simulink library "metux_library"  (R2025b)
settings: Solver=VariableStepAuto  StartTime=0.0  StopTime=10.0  RelTol=1e-3
values from neighbouring files (symbols this model uses):
  controllerGains = Simulink.Parameter(controllerGains)    [currentControllerInit.m]
  R = 287    [fluid_contants.m]
undefined symbols (not defined in the file or in its folder): b, bp, bv, DiscIntNeverNeededParam, fluid, Fs_max, J, Km, kp, L, omega_bandwidth, T_brk, T_c, valveAngle, valveFit
libraries: simulink x5, slpidlib x1, eeGeneralControl x1
settings Model: Creator=karadeli  LastModifiedBy=karadeli

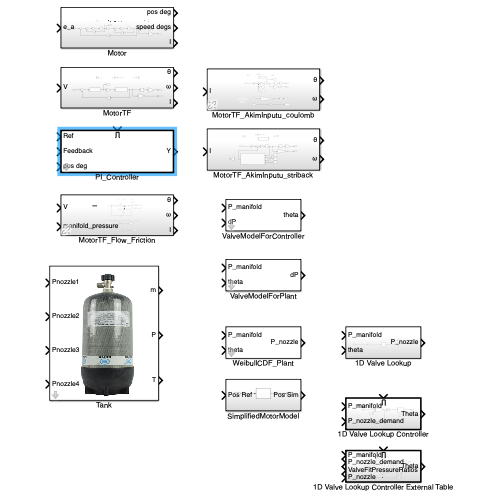
[thumbnail: Simulink's stored preview of the top-level diagram]
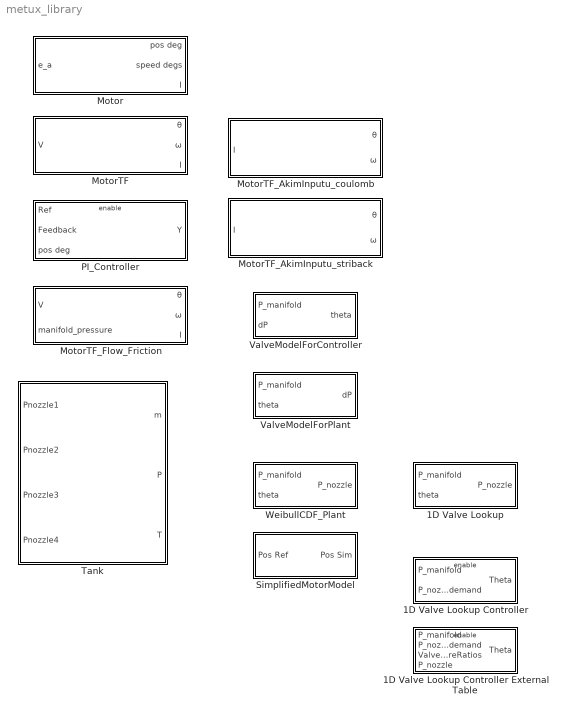
== system metux_library ==
  1D Valve Lookup : Subsystem
  1D Valve Lookup Controller : Subsystem
  1D Valve Lookup Controller External Table : Subsystem
  Motor : Subsystem
  MotorTF : Subsystem
  MotorTF_AkimInputu_coulomb : Subsystem  AncestorBlock=metux_library/MotorTF
  MotorTF_AkimInputu_striback : Subsystem
  MotorTF_Flow_Friction : Subsystem  AncestorBlock=metux_library/MotorTF
  PI_Controller : Subsystem  mask{Kp=1, Ki=1, SatMax=0, SatMin=0, Ts=1e-3, RateLimiterMax=0, RateLimiterMin=0}
  SimplifiedMotorModel : Subsystem
  Tank : Subsystem  mask{P0=300, T0=25, mdotGain=fluid.mdotGain, V=fluid.V, R=fluid.R, Cv=fluid.Cv, Patm=fluid.Patm}
      mask Display: image('Tank.png');
  ValveModelForController : Subsystem  mask{alpha=51.8534, C_max=0.9197}
  ValveModelForPlant : Subsystem  mask{C_max=0.9197, alpha=51.8534}
  WeibullCDF_Plant : Subsystem  mask{L=0.7772, tau=519.6652, n=1.5198}

== system metux_library/1D Valve Lookup ==
  P_manifold : Inport  Unit=psi
  theta : Inport  Port=2  Unit=deg
  1-D Lookup Table : Lookup_n-D  NumberOfTableDimensions=1  BreakpointsForDimension1=valveFit.angles  Table=valveFit.pressureRatios  InterpMethod=Linear Lagrange  ExtrapMethod=Clip  InternalRulePriority=Speed  RndMeth=Simplest
  Product1 : Product
  Saturation : Saturate  UpperLimit=5*360  LowerLimit=0
  P_nozzle : Outport  Unit=psi
  wires:
  1-D Lookup Table/1 -> Product1/2
  P_manifold/1 -> Product1/1
  Product1/1 -> P_nozzle/1
  theta/1 -> Saturation/1
  Saturation/1 -> 1-D Lookup Table/1

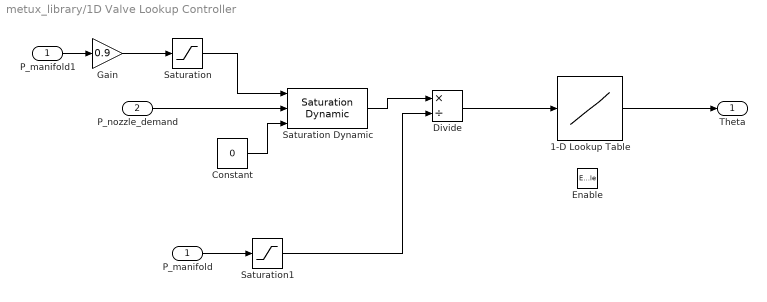
== system metux_library/1D Valve Lookup Controller ==
  P_manifold : Inport  Unit=psi
  P_nozzle_demand : Inport  Port=2  Unit=psi
  Enable : EnablePort
  1-D Lookup Table : Lookup_n-D  NumberOfTableDimensions=1  BreakpointsForDimension1=valveFit.pressureRatios  Table=valveFit.angles  InterpMethod=Linear Lagrange  ExtrapMethod=Clip  InternalRulePriority=Speed  RndMeth=Simplest
  Constant : Constant  Value=0
  Divide : Product  Inputs=*/
  Gain : Gain  Gain=0.9
  P_manifold1 : InportShadow  Unit=psi
  Saturation : Saturate  UpperLimit=5000  LowerLimit=15
  Saturation Dynamic : simulink/Discontinuities/Saturation Dynamic  OutMin=[]  OutMax=[]  OutDataTypeStr=Inherit: Same as second input  OutDataType=fixdt(1, 16)  OutScaling=2^-10  DoSatur=off
  Saturation1 : Saturate  UpperLimit=5000  LowerLimit=15
  Theta : Outport  Unit=deg
  wires:
  P_nozzle_demand/1 -> Saturation Dynamic/2
  1-D Lookup Table/1 -> Theta/1
  Saturation Dynamic/1 -> Divide/1
  Constant/1 -> Saturation Dynamic/3
  P_manifold1/1 -> Gain/1
  Gain/1 -> Saturation/1
  Saturation/1 -> Saturation Dynamic/1
  P_manifold/1 -> Saturation1/1
  Saturation1/1 -> Divide/2
  Divide/1 -> 1-D Lookup Table/1

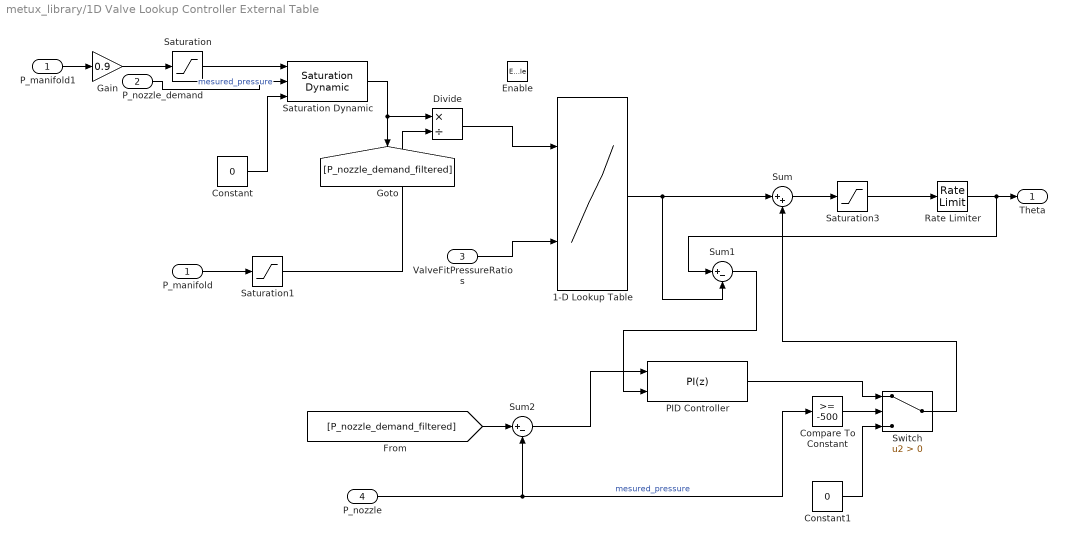
== system metux_library/1D Valve Lookup Controller External Table ==
  P_manifold : Inport  Unit=psi
  P_nozzle_demand : Inport  Port=2  Unit=psi
  ValveFitPressureRatios : Inport  Port=3  Unit=psi  PortDimensions=11
  P_nozzle : Inport  Port=4
  Enable : EnablePort
  1-D Lookup Table : Lookup_n-D  NumberOfTableDimensions=1  BreakpointsForDimension1Source=Input port  BreakpointsForDimension1=valveFit.pressureRatios  Table=[0 100 200 300 400 500 600 800 900 1100 1200 ]  InterpMethod=Linear Lagrange  ExtrapMethod=Clip  InternalRulePriority=Speed  RndMeth=Simplest
      settings: InputPortMap=u0,p5
  Compare To Constant : simulink/Logic and Bit Operations/Compare To Constant  relop=>=  const=-500  OutDataTypeStr=boolean
  Constant : Constant  Value=0
  Constant1 : Constant  Value=0
  Divide : Product  Inputs=*/
  Gain : Gain  Gain=0.9
  PID Controller : slpidlib/PID Controller  Controller=PI  Form=Parallel  TimeDomain=Discrete-time  UseExternalTs=off  SampleTime=-1  IntegratorMethod=Forward Euler  FilterMethod=Forward Euler  ControllerParametersSource=internal  P=controllerGains.pressure.Kp  I=controllerGains.pressure.Ki  UseKiTs=off  D=0  UseExternalDerivativeSource=off  N=100  UseFilter=on  TunerSelectOption=Transfer Function Based (PID Tuner App)  InitialConditionSource=internal  InitialConditionForIntegrator=0  InitialConditionForFilter=0  DifferentiatorICPrevScaledInput=0  ExternalReset=none  TrackingMode=on  Kt=100  LimitOutput=off  SatLimitsSource=internal  UpperSaturationLimit=200  LowerSaturationLimit=-200  LinearizeAsGain=on  AntiWindupMode=none  Kb=1  LimitIntegrator=off  UpperIntegratorSaturationLimit=200  LowerIntegratorSaturationLimit=-200  POutMin=[]  POutMax=[]  IOutMin=[]  IOutMax=[]  DOutMin=[]  DOutMax=[]  NOutMin=[]  NOutMax=[]  SumOutMin=[]  SumOutMax=[]  SaturationOutMin=[]  SaturationOutMax=[]  PParamMin=[]  PParamMax=[]  IParamMin=[]  IParamMax=[]  DParamMin=[]  DParamMax=[]  NParamMin=[]  NParamMax=[]  KbParamMin=[]  KbParamMax=[]  KtParamMin=[]  KtParamMax=[]  KbOutMin=[]  KbOutMax=[]  KtOutMin=[]  KtOutMax=[]  IntegratorOutMin=[]  IntegratorOutMax=[]  FilterOutMin=[]  FilterOutMax=[]  SumI1OutMin=[]  SumI1OutMax=[]  SumI2OutMin=[]  SumI2OutMax=[]  SumI3OutMin=[]  SumI3OutMax=[]  SumI4OutMin=[]  SumI4OutMax=[]  SumDOutMin=[]  SumDOutMax=[]  DifferentiatorOutMin=[]  DifferentiatorOutMax=[]  FilterDiffOutCoefMin=[]  FilterDiffOutCoefMax=[]  ReciprocalOutMin=[]  ReciprocalOutMax=[]  SumDenOutMin=[]  SumDenOutMax=[]  SumNumOutMin=[]  SumNumOutMax=[]  DivideOutMin=[]  DivideOutMax=[]  UdiffTsProdOutMin=[]  UdiffTsProdOutMax=[]  NTsProdOutMin=[]  NTsProdOutMax=[]  UintegralTsProdOutMin=[]  UintegralTsProdOutMax=[]  UngainTsProdOutMin=[]  UngainTsProdOutMax=[]  ClampingZeroOutDataTypeStr=Inherit: Inherit via back propagation  ClampingZeroOutMin=[]  ClampingZeroOutMax=[]  FilterDenConstantOutDataTypeStr=Inherit: Inherit via back propagation  FilterDenConstantOutMin=[]  FilterDenConstantOutMax=[]  PCopyOutDataTypeStr=Inherit: Inherit via back propagation  PCopyOutMin=[]  PCopyOutMax=[]  NCopyOutDataTypeStr=Inherit: Inherit via back propagation  NCopyOutMin=[]  NCopyOutMax=[]  IntegratorContinuousStateAttributes=''  IntegratorStateMustResolveToSignalObject=off  IntegratorRTWStateStorageClass=Auto  FilterContinuousStateAttributes=''  FilterStateMustResolveToSignalObject=off  FilterRTWStateStorageClass=Auto  ParallelPVariant=InternalParameters  IdealPVariant=Disabled  IVariant=InternalParameters  DVariant=Disabled  IntegratorVariant=Discrete  SatVariant=Disabled  AWVariant=Passthrough  PCopyVariant=Disabled  TRVariant=Enabled  FdbkBlocksVariant=Forward  IdealPFdbkVariant=Disabled  SatFdbkVariant=Disabled  DerivativeFilterVariant=Disabled  NVariant=Disabled  NCopyVariant=Disabled_SignalSpec  FilterICVariant=Disabled  IntegratorICVariant=InternalICs  ExternalResetVariant=Disabled  TRSumVariant=TrackingMode  SumFdbkVariant=Disabled  SumVariant=Sum_PI  TsampFilterVariant=InternalTs  TsampNgainVariant=Passthrough  TsampIntegralVariant=Disabled_SignalSpec  ExternalSaturationOutDataTypeStr=Inherit: Same as second input  DerivativeSourceVariant=Disabled  PreIntVariant=InternalPreInt
  P_manifold1 : InportShadow  Unit=psi
  Rate Limiter : RateLimiter  RisingSlewLimit=2000  FallingSlewLimit=-2000  SampleTimeMode=inherited
  Saturation : Saturate  UpperLimit=5000  LowerLimit=15
  Saturation Dynamic : simulink/Discontinuities/Saturation Dynamic  OutMin=[]  OutMax=[]  OutDataTypeStr=Inherit: Same as second input  OutDataType=fixdt(1, 16)  OutScaling=2^-10  DoSatur=off
  Saturation1 : Saturate  UpperLimit=5000  LowerLimit=15
  Saturation3 : Saturate  UpperLimit=1200  LowerLimit=0
  Sum : Sum  Inputs=|++
  Sum1 : Sum  Inputs=|+-
  Sum2 : Sum  Inputs=|+-
  Switch : Switch  Criteria=u2 > Threshold  SaturateOnIntegerOverflow=off  InputSameDT=off
  Theta : Outport  Unit=deg
  wires:
  Divide/1 -> 1-D Lookup Table/1
  Saturation1/1 -> Divide/2
  P_manifold/1 -> Saturation1/1
  Saturation/1 -> Saturation Dynamic/1
  Gain/1 -> Saturation/1
  P_manifold1/1 -> Gain/1
  Constant/1 -> Saturation Dynamic/3
  1-D Lookup Table/1 -> Sum1/2, Sum/1
  P_nozzle_demand/1 -> Saturation Dynamic/2  "mesured_pressure"
  ValveFitPressureRatios/1 -> 1-D Lookup Table/2
  P_nozzle/1 -> Compare To Constant/1, Sum2/2  "mesured_pressure"
  Saturation Dynamic/1 -> [P_nozzle_demand_filtered], Divide/1
  Sum2/1 -> PID Controller/1
  Saturation3/1 -> Rate Limiter/1
  Sum/1 -> Saturation3/1
  Switch/1 -> Sum/2
  Compare To Constant/1 -> Switch/2
  PID Controller/1 -> Switch/1
  Constant1/1 -> Switch/3
  [P_nozzle_demand_filtered] -> Sum2/1
  Rate Limiter/1 -> Sum1/1, Theta/1
  Sum1/1 -> PID Controller/2

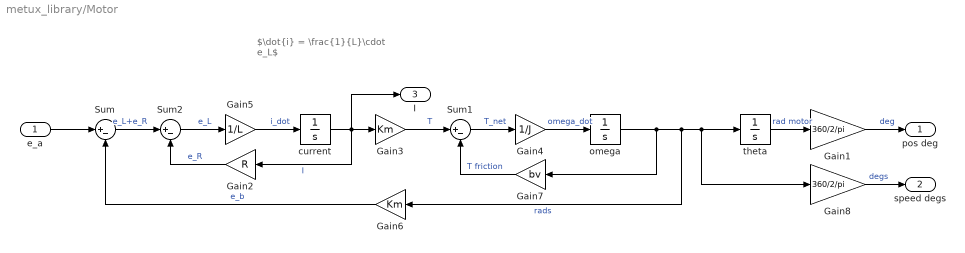
== system metux_library/Motor ==
  note: $\dot{i} = \frac{1}{L}\cdot e_L$
  e_a : Inport
  Gain1 : Gain  Gain=360/2/pi
  Gain2 : Gain  Gain=R
  Gain3 : Gain  Gain=Km
  Gain4 : Gain  Gain=1/J
  Gain5 : Gain  Gain=1/L
  Gain6 : Gain  Gain=Km
  Gain7 : Gain  Gain=bv
  Gain8 : Gain  Gain=360/2/pi
  Sum : Sum  Inputs=|+-
  Sum1 : Sum  Inputs=|+-
  Sum2 : Sum  Inputs=|+-
  current : Integrator
  omega : Integrator
  theta : Integrator  InitialCondition=valveAngle.Data(1)*13.7/180*pi  ZeroCross=off
  pos deg : Outport
  speed degs : Outport  Port=2
  I : Outport  Port=3
  wires:
  Sum1/1 -> Gain4/1  "T_net"
  theta/1 -> Gain1/1  "rad motor"
  current/1 -> Gain3/1, Gain2/1, I/1  "I"
  Sum/1 -> Sum2/1  "e_L+e_R"
  Gain5/1 -> current/1  "i_dot"
  Gain4/1 -> omega/1  "omega_dot"
  Gain2/1 -> Sum2/2  "e_R"
  Gain3/1 -> Sum1/1  "T"
  Gain6/1 -> Sum/2  "e_b"
  Gain7/1 -> Sum1/2  "T friction"
  Sum2/1 -> Gain5/1  "e_L"
  omega/1 -> theta/1, Gain8/1, Gain6/1, Gain7/1  "rads"
  e_a/1 -> Sum/1
  Gain1/1 -> pos deg/1  "deg"
  Gain8/1 -> speed degs/1  "degs"

== system metux_library/MotorTF ==
  note: $e_b = K_b\cdot\frac{d\theta}{dt}$
  note: $L_a\cdot\frac{di_a}{dt}+R_ai_a+e_b=e_a$
  note: $\frac{di}{dt} = \frac{1}{L}\cdot e_L$
  V : Inport  Unit=V
  Gain1 : Gain  Gain=360/2/pi
  Gain3 : Gain  Gain=Km
  Gain6 : Gain  Gain=Km
  Gain8 : Gain  Gain=360/2/pi
  Sum : Sum  Inputs=|+-
  current : TransferFcn  Denominator=[L R]  ContinuousStateAttributes='current'
  speed : TransferFcn  Denominator=[J bv]  ContinuousStateAttributes='speed'
  theta : Integrator  ZeroCross=off
  θ : Outport  Unit=deg
  ω : Outport  Port=2  Unit=deg/s
  I : Outport  Port=3  Unit=A
  wires:
  Gain1/1 -> θ/1  "deg"
  theta/1 -> Gain1/1  "rad motor"
  Gain8/1 -> ω/1  "degs"
  speed/1 -> theta/1, Gain8/1, Gain6/1  "rads"
  Gain3/1 -> speed/1  "T"
  current/1 -> Gain3/1, I/1  "I"
  Gain6/1 -> Sum/2  "e_b"
  Sum/1 -> current/1  "e_L+e_R"
  V/1 -> Sum/1

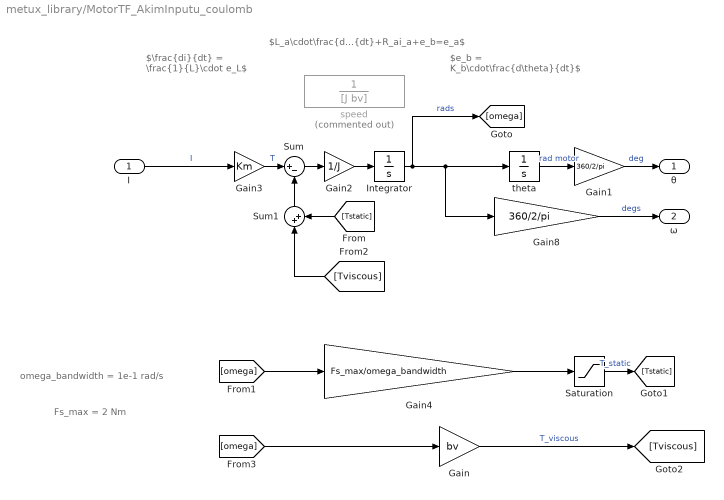
== system metux_library/MotorTF_AkimInputu_coulomb ==
  note: Fs_max = 2 Nm
  note: omega_bandwidth = 1e-1 rad/s
  note: $\frac{di}{dt} = \frac{1}{L}\cdot e_L$
  note: $L_a\cdot\frac{di_a}{dt}+R_ai_a+e_b=e_a$
  note: $e_b = K_b\cdot\frac{d\theta}{dt}$
  I : Inport  Unit=A
  Gain : Gain  Gain=bv
  Gain1 : Gain  Gain=360/2/pi
  Gain2 : Gain  Gain=1/J
  Gain3 : Gain  Gain=Km
  Gain4 : Gain  Gain=Fs_max/omega_bandwidth
  Gain8 : Gain  Gain=360/2/pi
  Integrator : Integrator
  Saturation : Saturate  UpperLimit=Fs_max  LowerLimit=-Fs_max  ZeroCross=off
  Sum : Sum  Inputs=|+-
  Sum1 : Sum  Inputs=|++
  speed : TransferFcn  Commented=on  Denominator=[J bv]  ContinuousStateAttributes='speed'
  theta : Integrator  ZeroCross=off
  θ : Outport  Unit=deg
  ω : Outport  Port=2  Unit=deg/s
  wires:
  I/1 -> Gain3/1  "I"
  Gain3/1 -> Sum/1  "T"
  Integrator/1 -> [omega], Gain8/1, theta/1  "rads"
  Gain8/1 -> ω/1  "degs"
  theta/1 -> Gain1/1  "rad motor"
  Gain1/1 -> θ/1  "deg"
  Sum/1 -> Gain2/1
  Gain2/1 -> Integrator/1
  [omega] -> Gain4/1
  Gain4/1 -> Saturation/1
  Sum1/1 -> Sum/2
  Saturation/1 -> [Tstatic]  "T_static"
  [Tstatic] -> Sum1/2
  Gain/1 -> [Tviscous]  "T_viscous"
  [Tviscous] -> Sum1/1
  [omega] -> Gain/1

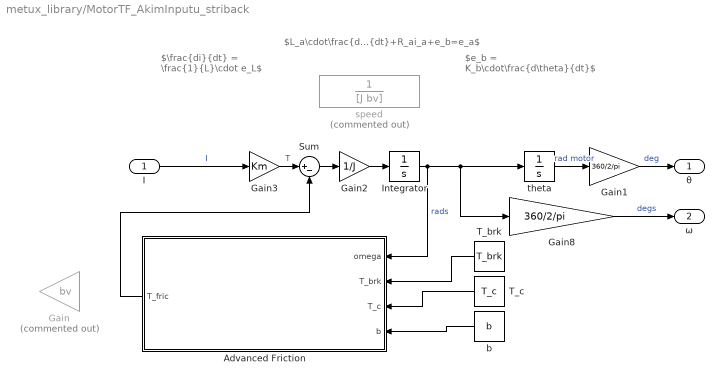
== system metux_library/MotorTF_AkimInputu_striback ==
  note: $e_b = K_b\cdot\frac{d\theta}{dt}$
  note: $L_a\cdot\frac{di_a}{dt}+R_ai_a+e_b=e_a$
  note: $\frac{di}{dt} = \frac{1}{L}\cdot e_L$
  I : Inport  Unit=A
  Advanced Friction : MATLAB Function  TreatAsAtomicUnit=on
  Gain : Gain  Commented=on  Gain=bv
  Gain1 : Gain  Gain=360/2/pi
  Gain2 : Gain  Gain=1/J
  Gain3 : Gain  Gain=Km
  Gain8 : Gain  Gain=360/2/pi
  Integrator : Integrator
  Sum : Sum  Inputs=|+-
  T_brk : Constant  Value=T_brk
  T_c : Constant  Value=T_c
  b : Constant  Value=b
  speed : TransferFcn  Commented=on  Denominator=[J bv]  ContinuousStateAttributes='speed'
  theta : Integrator  ZeroCross=off
  θ : Outport  Unit=deg
  ω : Outport  Port=2  Unit=deg/s
  wires:
  T_brk/1 -> Advanced Friction/2(T_brk)
  b/1 -> Advanced Friction/4(b)
  T_c/1 -> Advanced Friction/3(T_c)
  Gain2/1 -> Integrator/1
  Advanced Friction/1(T_fric) -> Sum/2
  Sum/1 -> Gain2/1
  Gain1/1 -> θ/1  "deg"
  theta/1 -> Gain1/1  "rad motor"
  Gain8/1 -> ω/1  "degs"
  Integrator/1 -> Advanced Friction/1(omega), theta/1, Gain8/1  "rads"
  Gain3/1 -> Sum/1  "T"
  I/1 -> Gain3/1  "I"

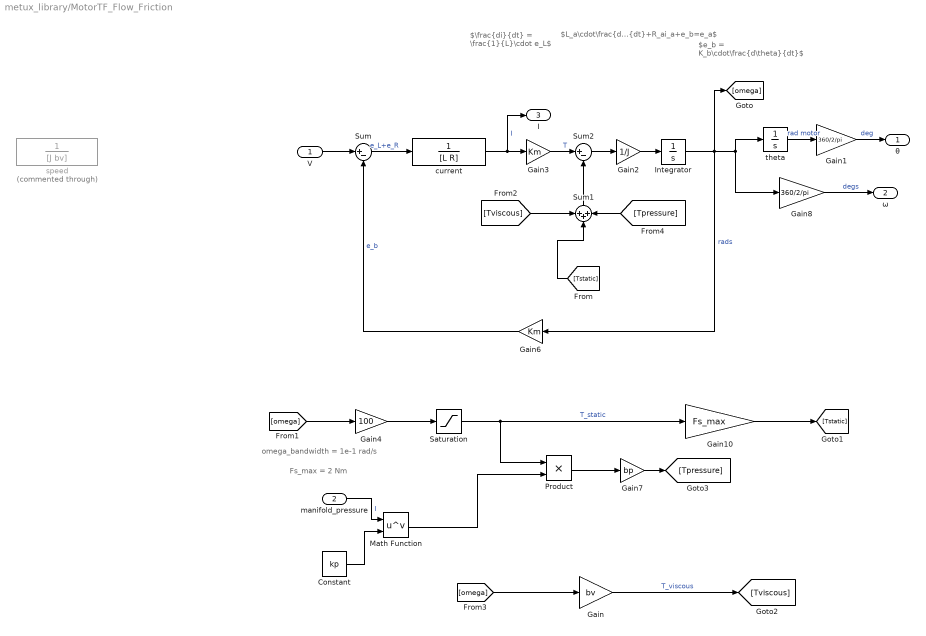
== system metux_library/MotorTF_Flow_Friction ==
  note: $\frac{di}{dt} = \frac{1}{L}\cdot e_L$
  note: $L_a\cdot\frac{di_a}{dt}+R_ai_a+e_b=e_a$
  note: $e_b = K_b\cdot\frac{d\theta}{dt}$
  note: Fs_max = 2 Nm
  note: omega_bandwidth = 1e-1 rad/s
  V : Inport  Unit=V
  manifold_pressure : Inport  Port=2
  Constant : Constant  Value=kp
  Gain : Gain  Gain=bv
  Gain1 : Gain  Gain=360/2/pi
  Gain10 : Gain  Gain=Fs_max
  Gain2 : Gain  Gain=1/J
  Gain3 : Gain  Gain=Km
  Gain4 : Gain  Gain=100
  Gain6 : Gain  Gain=Km
  Gain7 : Gain  Gain=bp
  Gain8 : Gain  Gain=360/2/pi
  Integrator : Integrator
  Math Function : Math  Operator=pow
  Product : Product
  Saturation : Saturate  UpperLimit=1  LowerLimit=-1
  Sum : Sum  Inputs=|+-
  Sum1 : Sum  Inputs=+++
  Sum2 : Sum  Inputs=|+-
  current : TransferFcn  Denominator=[L R]  ContinuousStateAttributes='current'
  speed : TransferFcn  Commented=through  Denominator=[J bv]  ContinuousStateAttributes='speed'
  theta : Integrator  ZeroCross=off
  θ : Outport  Unit=deg
  ω : Outport  Port=2  Unit=deg/s
  I : Outport  Port=3  Unit=A
  wires:
  V/1 -> Sum/1
  Sum/1 -> current/1  "e_L+e_R"
  Gain6/1 -> Sum/2  "e_b"
  current/1 -> I/1, Gain3/1  "I"
  Gain3/1 -> Sum2/1  "T"
  Integrator/1 -> Gain6/1, Gain8/1, theta/1, [omega]  "rads"
  Gain8/1 -> ω/1  "degs"
  theta/1 -> Gain1/1  "rad motor"
  Gain1/1 -> θ/1  "deg"
  [omega] -> Gain4/1
  Constant/1 -> Math Function/2
  Product/1 -> Gain7/1
  [omega] -> Gain/1
  Gain/1 -> [Tviscous]  "T_viscous"
  Saturation/1 -> Gain10/1, Product/1  "T_static"
  manifold_pressure/1 -> Math Function/1  "I"
  Gain10/1 -> [Tstatic]
  Gain7/1 -> [Tpressure]
  Math Function/1 -> Product/2
  Gain4/1 -> Saturation/1
  [Tstatic] -> Sum1/2
  [Tpressure] -> Sum1/3
  Sum1/1 -> Sum2/2
  [Tviscous] -> Sum1/1
  Sum2/1 -> Gain2/1
  Gain2/1 -> Integrator/1

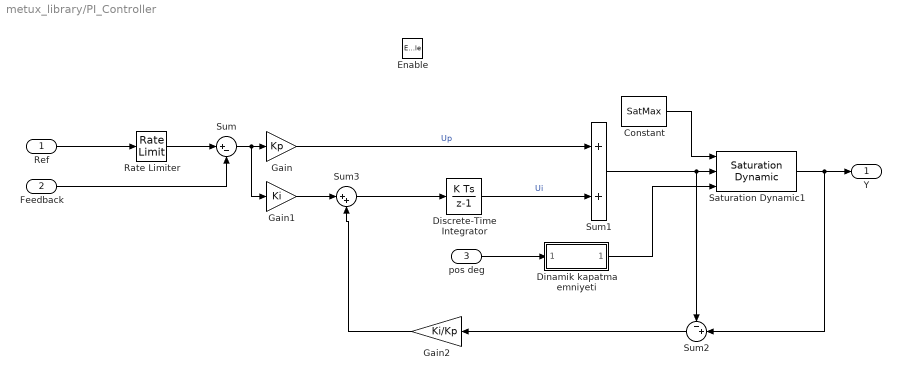
== system metux_library/PI_Controller ==
  Ref : Inport  SampleTime=Ts
  Feedback : Inport  Port=2  SampleTime=Ts
  pos deg : Inport  Port=3
  Enable : EnablePort  StatesWhenEnabling=reset
  Constant : Constant  Value=SatMax
  Dinamik kapatma emniyeti : Subsystem
  Discrete-Time Integrator : DiscreteIntegrator  SampleTime=Ts  LimitOutput=on  UpperSaturationLimit=SatMax  LowerSaturationLimit=SatMin  ICPrevOutput=DiscIntNeverNeededParam  ICPrevScaledInput=DiscIntNeverNeededParam
  Gain : Gain  Gain=Kp
  Gain1 : Gain  Gain=Ki
  Gain2 : Gain  Gain=Ki/Kp
  Rate Limiter : RateLimiter  RisingSlewLimit=RateLimiterMax  FallingSlewLimit=RateLimiterMin  SampleTimeMode=inherited
  Saturation Dynamic1 : simulink/Discontinuities/Saturation Dynamic  OutMin=[]  OutMax=[]  OutDataTypeStr=Inherit: Same as second input  OutDataType=fixdt(1, 16)  OutScaling=2^-10  DoSatur=off
  Sum : Sum  Inputs=|+-
  Sum1 : Sum
  Sum2 : Sum  Inputs=-+|
  Sum3 : Sum  Inputs=|++
  Y : Outport  SampleTime=Ts  OutputWhenDisabled=reset  InitialOutput=[0.0]
  wires:
  Saturation Dynamic1/1 -> Y/1, Sum2/2
  Discrete-Time Integrator/1 -> Sum1/2  "Ui"
  Gain1/1 -> Sum3/1
  Sum/1 -> Gain1/1, Gain/1
  Gain/1 -> Sum1/1  "Up"
  Feedback/1 -> Sum/2
  Sum1/1 -> Saturation Dynamic1/2, Sum2/1
  Ref/1 -> Rate Limiter/1
  Sum2/1 -> Gain2/1
  Gain2/1 -> Sum3/2
  Rate Limiter/1 -> Sum/1
  Constant/1 -> Saturation Dynamic1/1
  Sum3/1 -> Discrete-Time Integrator/1
  pos deg/1 -> Dinamik kapatma emniyeti/1(pos deg)
  Dinamik kapatma emniyeti/1(Lower Sat Limit) -> Saturation Dynamic1/3

== system metux_library/SimplifiedMotorModel ==
  Pos Ref : Inport  Unit=deg
  Second-Order Filter : eeGeneralControl/Second-Order Filter  FilterType=Low-pass  fn=20  Zeta=0.8  Ts=0  A0=0  Ph0=0  f0=0  b0=0
  Pos Sim : Outport  Unit=deg
  wires:
  Pos Ref/1 -> Second-Order Filter/1
  Second-Order Filter/1 -> Pos Sim/1

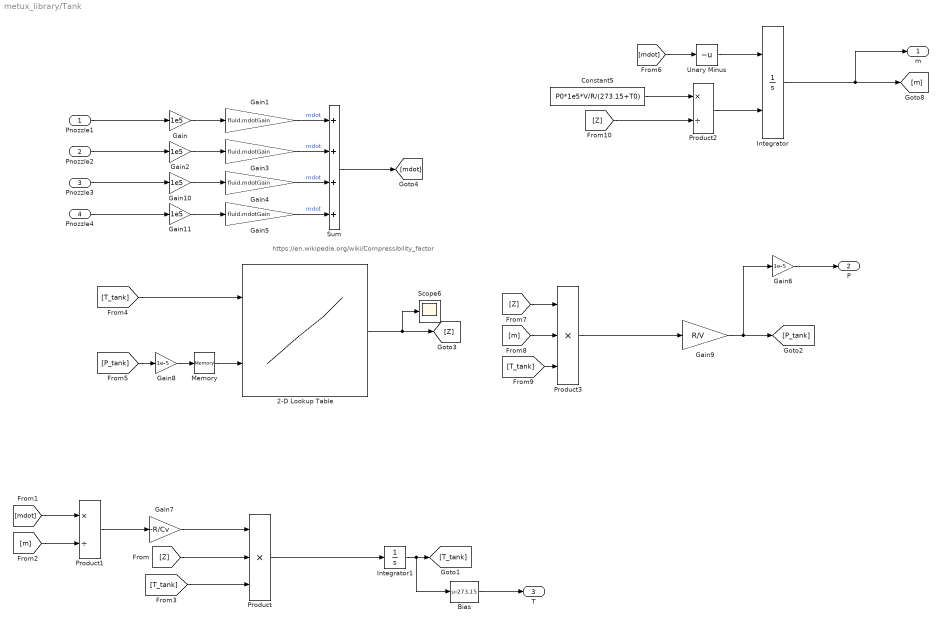
== system metux_library/Tank ==
  note: https://en.wikipedia.org/wiki/Compressibility_factor
  Pnozzle1 : Inport  Unit=bar
  Pnozzle2 : Inport  Port=2  Unit=bar
  Pnozzle3 : Inport  Port=3  Unit=bar
  Pnozzle4 : Inport  Port=4  Unit=bar
  2-D Lookup Table : Lookup_n-D  BreakpointsForDimension1=[75;80;90;100;120;140;160;180;200;250;300;350;400;450;500;600;800;1000]  BreakpointsForDimension2=[1;5;10;20;40;60;80;100;150;200;250;300;400;500]  Table=[0.0052 0.0260 0.0519 0.1036 0.2063 0.3082 0.4094 0.5099 0.7581 1.0125 0.0000 0.0000 0.0000 0.0000;0.0000 0.0250 0.0499 0.0995 0.1981 0.2958 0.3927 0.4887 0.7258 0.9588 1.1931 1.4139 0.0000 0.0000;0.9764 0.0236 0.0453 0.0940 0.1866 0.2781 0.3686 0.4681 0.6779 0.8929 1.1098 1.3110 1.7161 2.1105;0.9797 0.8872 0.0453 0.0900 0.1782 0.2635 0.3498 0.4337 0.6386 0.8377 1.0395 1.2227 1.5937 1.9536;0.9880 0.9373 0.8860 0.6730 0.1778 0.2557 0.3371 0.4132 0.5964 0.7720 0.9530 1.1076 1.5091 1.7366;0.9927 0.9614 0.9205 0.8297 0.5856 0.3313 0.3737 0.4340 0.5909 0.7699 0.9114 1.0393 1.3202 1.5903;0.9951 0.9748 0.9489 0.8954 0.7803 0.6603 0.5696 0.5489 0.6340 0.7564 0.8840 1.0105 1.2585 1.4970;0.9967 0.9832 0.9660 0.9314 0.8625 0.7977 0.7432 0.7084 0.7180 0.7986 0.9000 1.0068 1.2232 1.4361;0.9978 0.9886 0.9767 0.9539 0.9100 0.8701 0.8374 0.8142 0.8061 0.8549 0.9311 1.0185 1.2054 1.3944;0.9992 0.9957 0.9911 0.9822 0.9671 0.9549 0.9463 0.9411 0.9450 0.9713 1.0152 1.0702 1.1990 1.3392;0.9999 0.9987 0.9974 0.9950 0.9917 0.9901 0.9903 0.9930 1.0074 1.0326 1.0669 1.1089 1.2073 1.3163;1.0000 1.0002 1.0004 1.0014 1.0038 1.0075 1.0121 1.0183 1.0377 1.0635 1.0947 1.1303 1.2116 1.3015;1.0002 1.0012 1.0025 1.0046 1.0100 1.0159 1.0229 1.0312 1.0533 1.0795 1.1087 1.1411 1.2117 1.2890;1.0003 1.0016 1.0034 1.0063 1.0133 1.0210 1.0287 1.0374 1.0614 1.0913 1.1183 1.1463 1.2090 1.2778;1.0003 1.0020 1.0034 1.0074 1.0151 1.0234 1.0323 1.0410 1.0650 1.0913 1.1183 1.1463 1.2051 1.2667;1.0004 1.0022 1.0039 1.0081 1.0164 1.0253 1.0340 1.0434 1.0678 1.0920 1.1172 1.1427 1.1947 1.2475;1.0004 1.0020 1.0038 1.0077 1.0157 1.0240 1.0321 1.0408 1.0621 1.0844 1.1061 1.1283 1.1720 1.2150;1.0004 1.0018 1.0037 1.0068 1.0142 1.0215 1.0290 1.0365 1.0556 1.0744 1.0948 1.1131 1.1515 1.1889]  InternalRulePriority=Speed  RndMeth=Simplest
      settings: InputPortMap=u0,u1
  Bias : Bias  Bias=-273.15  SaturateOnIntegerOverflow=off
  Constant5 : Constant  Value=P0*1e5*V/R/(273.15+T0)
  Gain{,2,10..11} (4 alike) : Gain  Gain=1e5
  Gain{1,3..5} (4 alike) : Gain  Gain=fluid.mdotGain
  Gain6 : Gain  Gain=1e-5
  Gain7 : Gain  Gain=-R/Cv
  Gain8 : Gain  Gain=1e-5
  Gain9 : Gain  Gain=R/V
  Integrator : Integrator  InitialConditionSource=external  InitialCondition=3  LimitOutput=on  UpperSaturationLimit=5  LowerSaturationLimit=Patm*V/R/100
  Integrator1 : Integrator  InitialCondition=T0+273.15  LowerSaturationLimit=0
  Memory : Memory  InitialCondition=P0
  Product : Product  Inputs=3
  Product1 : Product  Inputs=*/
  Product2 : Product  Inputs=*/
  Product3 : Product  Inputs=3
  Scope6 : Scope
      settings: ActiveDisplayYMinimum=0.8767629134747118  ActiveDisplayYMaximum=1.1251537258363551  DataLoggingVariableName=ScopeData19
  Sum : Sum  Inputs=4
  Unary Minus : UnaryMinus
  m : Outport  Unit=kg
  P : Outport  Port=2  Unit=bar
  T : Outport  Port=3  Unit=°C
  wires:
  Gain1/1 -> Sum/1  "mdot"
  Pnozzle1/1 -> Gain/1
  Unary Minus/1 -> Integrator/1
  Integrator/1 -> m/1, [m]
  [mdot] -> Unary Minus/1
  Constant5/1 -> Product2/1
  Pnozzle2/1 -> Gain2/1
  Pnozzle3/1 -> Gain10/1
  Pnozzle4/1 -> Gain11/1
  Gain5/1 -> Sum/4  "mdot"
  Gain4/1 -> Sum/3  "mdot"
  Gain3/1 -> Sum/2  "mdot"
  Sum/1 -> [mdot]
  Bias/1 -> T/1
  Gain6/1 -> P/1
  Gain7/1 -> Product/1
  Product/1 -> Integrator1/1
  Product1/1 -> Gain7/1
  [m] -> Product1/2
  Integrator1/1 -> Bias/1, [T_tank]
  [mdot] -> Product1/1
  [Z] -> Product/2
  [T_tank] -> Product/3
  Gain8/1 -> Memory/1
  2-D Lookup Table/1 -> [Z], Scope6/1
  [T_tank] -> 2-D Lookup Table/1
  [P_tank] -> Gain8/1
  Memory/1 -> 2-D Lookup Table/2
  Product3/1 -> Gain9/1
  Gain9/1 -> Gain6/1, [P_tank]
  [Z] -> Product3/1
  [m] -> Product3/2
  [T_tank] -> Product3/3
  Product2/1 -> Integrator/2
  [Z] -> Product2/2
  Gain/1 -> Gain1/1
  Gain2/1 -> Gain3/1
  Gain10/1 -> Gain4/1
  Gain11/1 -> Gain5/1

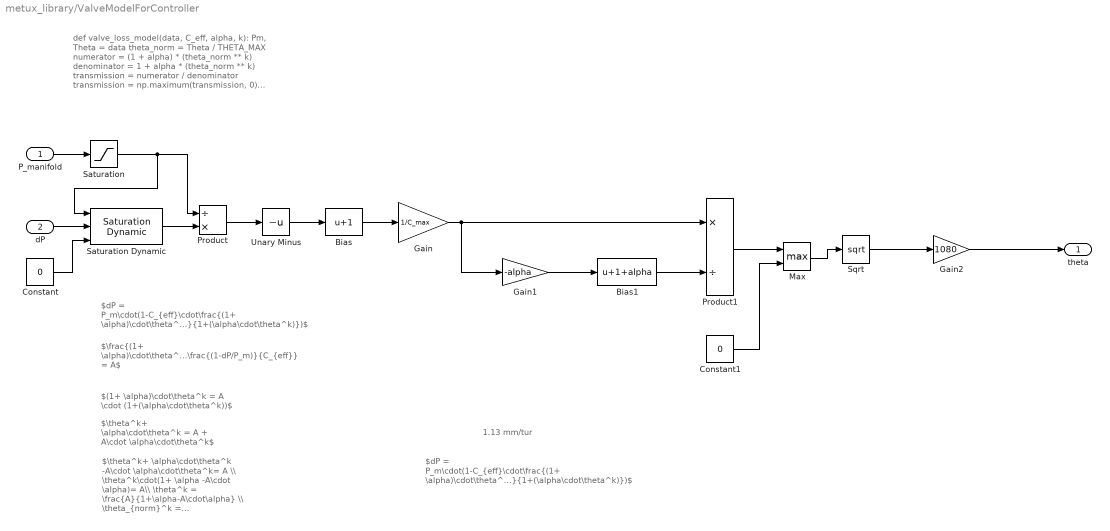
== system metux_library/ValveModelForController ==
  note: 1.13 mm/tur
  note: $dP = P_m\cdot(1-C_{eff}\cdot\frac{(1+ \alpha)\cdot\theta^k}{1+(\alpha\cdot\theta^k)})$
  note: def valve_loss_model(data, C_eff, alpha, k):
      |     Pm, Theta = data
      |     theta_norm = Theta / THETA_MAX
      |
      |     numerator = (1 + alpha) * (theta_norm ** k)
      |     denominator = 1 + alpha * (theta_norm ** k)
      |     transmission = numerator / denominator
      |     transmission = np.maximum(transmission, 0)
      |
      |     return Pm * (1 - C_eff * transmission)
  note: $\frac{(1+ \alpha)\cdot\theta^k}{1+(\alpha\cdot\theta^k)}=\frac{(1-dP/P_m)}{C_{eff}} = A$
  note: $(1+ \alpha)\cdot\theta^k = A \cdot (1+(\alpha\cdot\theta^k))$
  note: $\theta^k+ \alpha\cdot\theta^k = A + A\cdot \alpha\cdot\theta^k$
  note: $\theta^k+ \alpha\cdot\theta^k -A\cdot \alpha\cdot\theta^k= A \\ \theta^k\cdot(1+ \alpha -A\cdot \alpha)= A\\ \theta^k = \frac{A}{1+\alpha-A\cdot\alpha} \\ \theta_{norm}^k = \frac{\frac{(1-dP/P_m)}{C_{eff}}}{1+\alpha-(\frac{(1-dP/P_m)}{C_{eff}})\cdot\alpha}$
  note: $dP = P_m\cdot(1-C_{eff}\cdot\frac{(1+ \alpha)\cdot\theta^k}{1+(\alpha\cdot\theta^k)})$
  P_manifold : Inport
  dP : Inport  Port=2
  Bias : Bias  Bias=1  SaturateOnIntegerOverflow=off
  Bias1 : Bias  Bias=1+alpha  SaturateOnIntegerOverflow=off
  Constant : Constant  Value=0
  Constant1 : Constant  Value=0  OutDataTypeStr=single
  Gain : Gain  Gain=1/C_max
  Gain1 : Gain  Gain=-alpha
  Gain2 : Gain  Gain=1080
  Max : MinMax  Function=max  Inputs=2
  Product : Product  Inputs=/*
  Product1 : Product  Inputs=*/
  Saturation : Saturate  UpperLimit=5000  LowerLimit=0
  Saturation Dynamic : simulink/Discontinuities/Saturation Dynamic  OutMin=[]  OutMax=[]  OutDataTypeStr=Inherit: Same as second input  OutDataType=fixdt(1, 16)  OutScaling=2^-10  DoSatur=off
  Sqrt : Sqrt  OutputSignalType=real
  Unary Minus : UnaryMinus
  theta : Outport
  wires:
  P_manifold/1 -> Saturation/1
  Saturation/1 -> Saturation Dynamic/1, Product/1
  dP/1 -> Saturation Dynamic/2
  Constant/1 -> Saturation Dynamic/3
  Saturation Dynamic/1 -> Product/2
  Product/1 -> Unary Minus/1
  Unary Minus/1 -> Bias/1
  Bias/1 -> Gain/1
  Gain/1 -> Gain1/1, Product1/1
  Gain1/1 -> Bias1/1
  Bias1/1 -> Product1/2
  Max/1 -> Sqrt/1
  Sqrt/1 -> Gain2/1
  Gain2/1 -> theta/1
  Product1/1 -> Max/1
  Constant1/1 -> Max/2

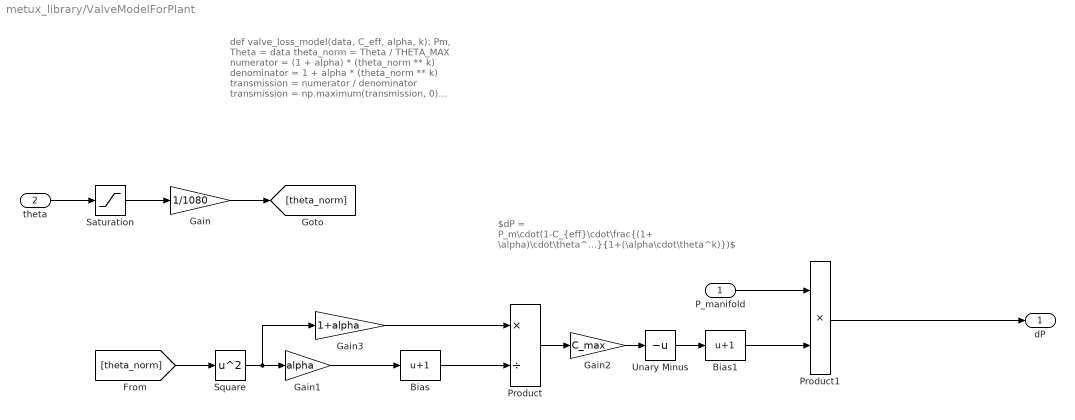
== system metux_library/ValveModelForPlant ==
  note: def valve_loss_model(data, C_eff, alpha, k):
      |     Pm, Theta = data
      |     theta_norm = Theta / THETA_MAX
      |
      |     numerator = (1 + alpha) * (theta_norm ** k)
      |     denominator = 1 + alpha * (theta_norm ** k)
      |     transmission = numerator / denominator
      |     transmission = np.maximum(transmission, 0)
      |
      |     return Pm * (1 - C_eff * transmission)
  note: $dP = P_m\cdot(1-C_{eff}\cdot\frac{(1+ \alpha)\cdot\theta^k}{1+(\alpha\cdot\theta^k)})$
  P_manifold : Inport  Unit=psi
  theta : Inport  Port=2  Unit=deg
  Bias : Bias  Bias=1  SaturateOnIntegerOverflow=off
  Bias1 : Bias  Bias=1  SaturateOnIntegerOverflow=off
  Gain : Gain  Gain=1/1080
  Gain1 : Gain  Gain=alpha
  Gain2 : Gain  Gain=C_max
  Gain3 : Gain  Gain=1+alpha
  Product : Product  Inputs=*/
  Product1 : Product
  Saturation : Saturate  UpperLimit=5*360  LowerLimit=0
  Square : Math  Operator=square
  Unary Minus : UnaryMinus
  dP : Outport  Unit=psi
  wires:
  Gain/1 -> [theta_norm]
  Square/1 -> Gain1/1, Gain3/1
  Gain1/1 -> Bias/1
  Bias/1 -> Product/2
  Product/1 -> Gain2/1
  Gain2/1 -> Unary Minus/1
  Unary Minus/1 -> Bias1/1
  Bias1/1 -> Product1/2
  P_manifold/1 -> Product1/1
  Product1/1 -> dP/1
  theta/1 -> Saturation/1
  [theta_norm] -> Square/1
  Gain3/1 -> Product/1
  Saturation/1 -> Gain/1

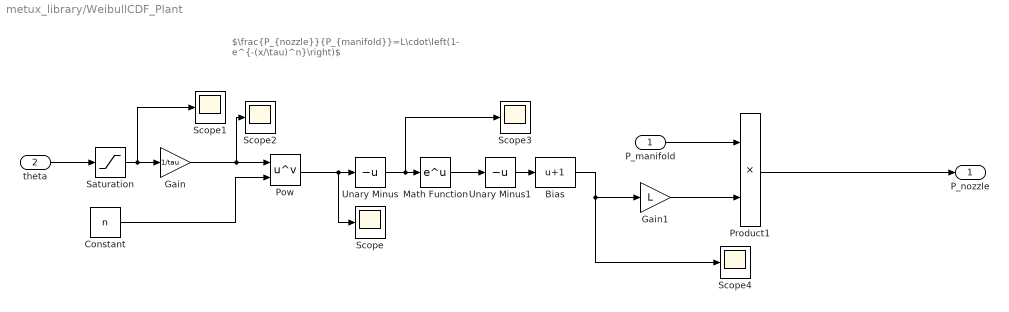
== system metux_library/WeibullCDF_Plant ==
  note: $\frac{P_{nozzle}}{P_{manifold}}=L\cdot\left(1- e^{-(x/\tau)^n}\right)$
  P_manifold : Inport  Unit=psi
  theta : Inport  Port=2  Unit=deg
  Bias : Bias  Bias=1  SaturateOnIntegerOverflow=off
  Constant : Constant  Value=n
  Gain : Gain  Gain=1/tau
  Gain1 : Gain  Gain=L
  Math Function : Math
  Pow : Math  Operator=pow  SignedPower=on  RndMeth=Zero
  Product1 : Product
  Saturation : Saturate  UpperLimit=5*360  LowerLimit=0
  Scope{,1..4} (5 alike) : Scope
      Scope2 settings: DataLoggingVariableName=ScopeData2
      Scope3 settings: DataLoggingVariableName=ScopeData3
      Scope4 settings: DataLoggingVariableName=ScopeData4
  Unary Minus : UnaryMinus
  Unary Minus1 : UnaryMinus
  P_nozzle : Outport  Unit=psi
  wires:
  theta/1 -> Saturation/1
  Product1/1 -> P_nozzle/1
  P_manifold/1 -> Product1/1
  Saturation/1 -> Scope1/1, Gain/1
  Gain/1 -> Scope2/1, Pow/1
  Constant/1 -> Pow/2
  Pow/1 -> Scope/1, Unary Minus/1
  Unary Minus/1 -> Scope3/1, Math Function/1
  Math Function/1 -> Unary Minus1/1
  Unary Minus1/1 -> Bias/1
  Bias/1 -> Scope4/1, Gain1/1
  Gain1/1 -> Product1/2

== system metux_library/PI_Controller/Dinamik kapatma emniyeti ==
  pos deg : Inport
  Constant1 : Constant  Value=SatMin  OutDataTypeStr=single
  Constant2 : Constant  Value=-2  OutDataTypeStr=single
  Constant3 : Constant  Value=-1.4  OutDataTypeStr=single
  Switch : Switch  Criteria=u2 > Threshold  Threshold=50  SaturateOnIntegerOverflow=off  InputSameDT=off
  Switch1 : Switch  Criteria=u2 > Threshold  Threshold=10  SaturateOnIntegerOverflow=off  InputSameDT=off
  Lower Sat Limit : Outport
  wires:
  Constant2/1 -> Switch1/1
  pos deg/1 -> Switch/2, Switch1/2
  Constant3/1 -> Switch1/3
  Switch1/1 -> Switch/3
  Switch/1 -> Lower Sat Limit/1
  Constant1/1 -> Switch/1

== matlab function metux_library/MotorTF_AkimInputu_striback/Advanced Friction ==
  data: omega input; T_brk input; T_fric output; T_c input; b input
function T_fric = advanced_friction(omega, T_brk, T_c, b)
% GELİŞMİŞ SÜRTÜNME MODELİ (Stribeck + Coulomb + Viscous)
% Bu model, kalkış anındaki zorlanmayı (T_brk) ve 
% hareket halindeki sürtünmeyi (T_c) ayrı ayrı hesaplar.

% Girişler:
%   omega : Hız (rad/s)
%   T_brk : Statik (Breakaway) Sürtünme Torku (Kalkış Zorluğu)
%   T_c   : Kinetik (Coulomb) Sürtünme Torku (Hareket Direnci)
%   b     : Viskoz Sürtünme (Hızla artan direnç)

    % --- Parametreler (Sabit Tutulacak) ---
    % w_st: Stribeck Hızı. Sürtünmenin T_brk'dan T_c'ye düştüğü hız.
    % Vana sistemleri için bu genelde düşüktür.
    w_st = 0.5;  % rad/s (Bunu estimate etme, sabit kalsın)
    
    % w_smooth: Sıfır geçiş yumuşatması (Zero-crossing)
    w_smooth = 0.05;

    % --- 1. Stribeck Etkisi (Exponential Decay) ---
    % Hız sıfırken (T_brk - T_c) kadar ek yük bindirir, hızlanınca yok olur.
    % Formül: (T_break - T_coulomb) * exp(-(w/w_st)^2)
    stribeck_effect = (T_brk - T_c) * exp(-(omega / w_st).^2);

    % --- 2. Toplam Sürtünme Katsayısı ---
    % Statik ve Kinetik sürtünmenin anlık toplamı
    F_total_coeff = T_c + stribeck_effect;

    % --- 3. Yön ve Viskozite ---
    % Tanh ile yön verilir + Viskoz terim eklenir
    T_fric = F_total_coeff * tanh(omega / w_smooth) + (b * omega);
    
end
